simulink model "SymmetricInterpolationFIR"  (R2024a)
settings: Solver=VariableStepAuto  StartTime=0.0  StopTime=300E-9  RelTol=1e-3
InitFcn:
  | coef=[-58,15,80,95,52,-27,-89,-96,-43,38,97,95,32,-53,-104,-90,-18,67,109,83,1,-80,-111,-69,16,94,109,54,-38,-106,-104,-32,62,117,95,7,-89,-127,-80,23,117,134,60,-60,-148,-139,-35,102,179,140,1,-150,-213,-137,38,205,249,130,-89,-269,-286,-117,146,337,323,97,-216,-415,-362,-69,295,501,402,34,-390,-598,-440,13,497,704,479,-71,-621,-824,-517,143,766,955,554,-232,-935,-1106,-589,341,1132,1275,623,-477,-1369,-1472,-655,646,1652,1703,683,-859,-2000,-1983,-710,1134,2441,2334,734,-1501,-3026,-2794,-756,2016,3845,3445,771,-2793,-5097,-4460,-785,4114,7301,6322,795,-6901,-12353,-11074,-800,17016,37340,53412,59511,53412,37340,17016,-800,-11074,-12353,-6901,795,6322,7301,4114,-785,-4460,-5097,-2793,771,3445,3845,2016,-756,-2794,-3026,-1501,734,2334,2441,1134,-710,-1983,-2000,-859,683,1703,1652,646,-655,-1472,-1369,-477,623,1275,1132,341,-589,-1106,-935,-232,554,955,766,143,-517,-824,-621,-71,479,704,497,13,-440,-598,-390,34,402,501,295,-69,-362,-415,-216,97,323,337,146,-117,-286,-269,-89,130,249,205,38,-137,-213,-150,1,140,179,102,-35,-139,-148,-60,60,134,117,23,-80,-127,-89,7,95,117,62,-32,-104,-106,-38,54,109,94,16,-69,-111,-80,1,83,109,67,-18,-90,-104,-53,32,95,97,38,-43,-96,-89,-27,52,95,80,15,-58;
  |        10,35,36,11,-23,-40,-29,4,35,41,18,-20,-45,-39,-4,36,52,31,-13,-51,-54,-20,31,63,52,5,-48,-69,-43,14,63,69,28,-33,-73,-62,-7,52,76,46,-17,-69,-72,-23,45,81,59,-8,-73,-87,-36,45,98,83,4,-85,-119,-69,35,123,131,45,-80,-158,-131,-10,126,183,117,-34,-168,-193,-86,85,202,183,36,-140,-220,-145,34,193,214,76,-124,-239,-176,30,233,272,97,-181,-359,-280,35,382,498,254,-232,-638,-648,-181,507,958,803,46,-881,-1353,-958,175,1383,1842,1107,-514,-2062,-2461,-1246,1032,3006,3282,1368,-1842,-4413,-4475,-1468,3226,6794,6517,1542,-6108,-12043,-11443,-1589,16342,37236,53942,60315,53942,37236,16342,-1589,-11443,-12043,-6108,1542,6517,6794,3226,-1468,-4475,-4413,-1842,1368,3282,3006,1032,-1246,-2461,-2062,-514,1107,1842,1383,175,-958,-1353,-881,46,803,958,507,-181,-648,-638,-232,254,498,382,35,-280,-359,-181,97,272,233,30,-176,-239,-124,76,214,193,34,-145,-220,-140,36,183,202,85,-86,-193,-168,-34,117,183,126,-10,-131,-158,-80,45,131,123,35,-69,-119,-85,4,83,98,45,-36,-87,-73,-8,59,81,45,-23,-72,-69,-17,46,76,52,-7,-62,-73,-33,28,69,63,14,-43,-69,-48,5,52,63,31,-20,-54,-51,-13,31,52,36,-4,-39,-45,-20,18,41,35,4,-29,-40,-23,11,36,35,10;
  |        25,21,1,-21,-29,-13,13,31,25,1,-25,-33,-16,13,33,28,2,-26,-35,-16,15,35,28,-2,-31,-36,-13,21,42,30,-7,-40,-45,-15,28,52,37,-6,-47,-53,-21,29,57,42,-5,-49,-55,-19,35,62,40,-15,-61,-61,-11,51,78,46,-26,-84,-81,-16,66,103,64,-24,-99,-101,-28,68,115,73,-26,-106,-104,-18,88,128,63,-60,-147,-122,7,149,188,83,-103,-231,-197,-7,205,284,155,-98,-293,-278,-53,220,332,186,-115,-335,-284,22,350,410,104,-376,-641,-403,264,904,972,253,-885,-1644,-1322,120,1866,2662,1662,-852,-3402,-4110,-1964,2238,6000,6443,2202,-5207,-11536,-11669,-2354,15609,37069,54456,61128,54456,37069,15609,-2354,-11669,-11536,-5207,2202,6443,6000,2238,-1964,-4110,-3402,-852,1662,2662,1866,120,-1322,-1644,-885,253,972,904,264,-403,-641,-376,104,410,350,22,-284,-335,-115,186,332,220,-53,-278,-293,-98,155,284,205,-7,-197,-231,-103,83,188,149,7,-122,-147,-60,63,128,88,-18,-104,-106,-26,73,115,68,-28,-101,-99,-24,64,103,66,-16,-81,-84,-26,46,78,51,-11,-61,-61,-15,40,62,35,-19,-55,-49,-5,42,57,29,-21,-53,-47,-6,37,52,28,-15,-45,-40,-7,30,42,21,-13,-36,-31,-2,28,35,15,-16,-35,-26,2,28,33,13,-16,-33,-25,1,25,31,13,-13,-29,-21,1,21,25;
  |        17,0,-17,-21,-8,12,22,14,-7,-21,-19,0,19,23,7,-16,-26,-15,9,27,24,0,-24,-29,-10,17,31,20,-9,-29,-26,0,27,32,9,-23,-38,-22,14,40,34,0,-36,-43,-16,26,46,29,-12,-44,-40,0,42,49,14,-36,-59,-33,23,64,55,0,-59,-72,-27,41,77,50,-20,-74,-66,0,70,83,23,-64,-105,-59,43,120,104,0,-112,-140,-56,77,151,102,-34,-146,-133,0,146,172,43,-149,-237,-129,114,301,262,0,-296,-385,-171,197,427,316,-69,-411,-400,0,466,552,76,-654,-997,-482,716,1743,1607,0,-2228,-3420,-2217,1249,4986,6105,2736,-4234,-10850,-11747,-3086,14817,36834,54947,61945,54947,36834,14817,-3086,-11747,-10850,-4234,2736,6105,4986,1249,-2217,-3420,-2228,0,1607,1743,716,-482,-997,-654,76,552,466,0,-400,-411,-69,316,427,197,-171,-385,-296,0,262,301,114,-129,-237,-149,43,172,146,0,-133,-146,-34,102,151,77,-56,-140,-112,0,104,120,43,-59,-105,-64,23,83,70,0,-66,-74,-20,50,77,41,-27,-72,-59,0,55,64,23,-33,-59,-36,14,49,42,0,-40,-44,-12,29,46,26,-16,-43,-36,0,34,40,14,-22,-38,-23,9,32,27,0,-26,-29,-9,20,31,17,-10,-29,-24,0,24,27,9,-15,-26,-16,7,23,19,0,-19,-21,-7,14,22,12,-8,-21,-17,0,17];
  | coef=coef';
  | H0=coef(1:4:273,:);H0=H0(:);
  | H1=coef(2:4:273,:);H1=H1(:);
  | H2=coef(3:4:273,:);H2=H2(:);
  | H3=coef(4:4:273,:);H3=H3(:);
  | H1PH3=H1+H3;
  | H1MH3=H1-H3;
undefined symbols (not defined in the file): S, vsva2197, xcvc1902
libraries: hdlBasic x29, hdlDSPIP x8, hdlUtilities x1, dspsrcs4 x1, dspsigops x1, vmcUtilities x1
settings Model: Creator=admin  LastModifiedBy=sdegala
settings SolverCC: AlgebraicLoopSolver=TrustRegion
settings DataIOCC: ReturnWorkspaceOutputs=off
settings DebuggingCC: UnconnectedInputMsg=warning  UnconnectedOutputMsg=warning  UnconnectedLineMsg=warning  ArithmeticOperatorsInVariantConditions=warning
settings ModelReferenceCC: EnableRefExpFcnMdlSchedulingChecks=on
settings SFSimCC: SimUseLocalCustomCode=off  CustomCodeUndefinedFunction=UseInterfaceOnly
settings RTWCC: RTWUseLocalCustomCode=off  GPUComputeCapability=3.5  DLArmComputeVersion=19.05
settings CodeAppCC: StateflowObjectComments=on

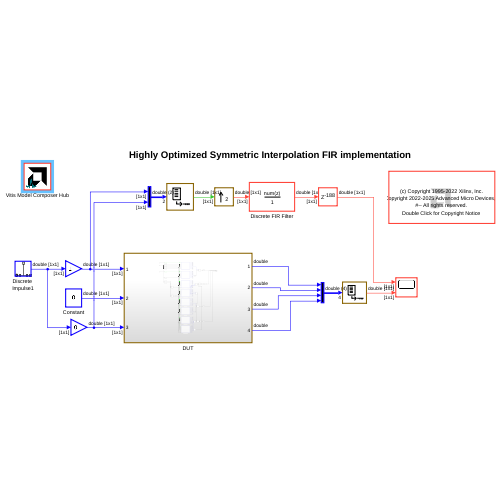
[thumbnail: Simulink's stored preview of the top-level diagram]
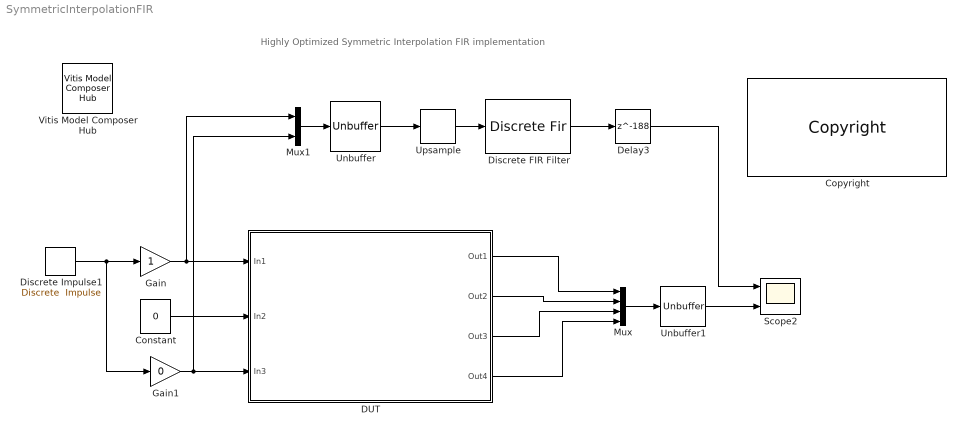
== system SymmetricInterpolationFIR ==
  note: Highly Optimized Symmetric Interpolation FIR implementation
  Constant : Constant  Value=0  VectorParams1D=off  SampleTime=-1
  Copyright : hdlUtilities/Copyright  copyrighttext="(c) Copyright 1995-2022 Xilinx, Inc. <br>(c) Copyright 2022-2025 Advanced Micro Devices, Inc. All rights reserved.<br><br>This document  contains proprietary, confidential information that may be used, copied and/or disclosed only as authorized by a valid licensing agreement with Advanced Micro Devices, Inc. This copyright notice must be retained on all authorized copies.<br><br> This code is provided \"as is\". Advanced Micro Devices, Inc. makes, and the end user receives, no warranties or conditions, express, implied, statutory or otherwise, and Advanced Micro Devices, Inc. specifically disclaims any implied warranties of merchantability, <br>non-infringement, or fitness for a particular purpose."  block_type=copyright
  DUT : Subsystem
  Delay3 : Delay  DelayLength=188
  Discrete Impulse1 : dspsrcs4/Discrete  Impulse  Delay=10  SampleTime=-1  FrameSample=1  OutputFrames=off  dataType=double  isSigned=on  wordLen=16  udDataType=sfix(16)  fracBitsMode=Best precision  numFracBits=15  OutDataTypeStr=double  LastOutDataTypeStr=double
  Discrete FIR Filter : DiscreteFir  Coefficients=coef(:,1)'  InputProcessing=Columns as channels (frame based)
  Gain : Gain
  Gain1 : Gain  Gain=0
  Mux : Mux
  Mux1 : Mux  Inputs=2
  Scope2 : Scope  NumInputPorts=2
  Unbuffer : Unbuffer
  Unbuffer1 : Unbuffer
  Upsample : dspsigops/Upsample  FactorSource=Dialog parameter  N=2  Nmax=16  phase=0  RateOptions=Allow multirate processing  ic=0  mode=Unused parameter value
  Vitis Model Composer Hub : vmcUtilities/Vitis Model Composer Hub  Tag=genX  CodeGeneration=off  SubsystemName=DUT  BlockHierPath=SymmetricInterpolationFIR/DUT  CompilationType=HDLCompilation  SubsystemType=HDLNode  ExportTypeV2=IP Catalog  StartColumn=1  NumberOfColumns=1  TargetDirectory=./netlist  exportDesign=on  analyzeDesign=off  validateDesignOnHw=off  ExportType=System Generator  IpVendor=xilinx.com  IpLibrary=hls  IpVersion=1.0  IpHWLanguage=Verilog  AieCompilerOptions={}  AieSimulatorOptions={}  CreateTestbench=off  TestbenchStackSize=10  RunRtlSim=off  RunCSim=off  RunAieSim=off  AieSimTimeout=50000  RunAieSimProfiling=off  LaunchVitisAnalyzer=off  PlotOutput=off  RunX86Sim=off  X86SimTimeout=10  GenHwImage=off  GenLibadfXo=off  GenHwValidationCode=off  PlatformType=Specify Platform  Platform=/proj/xbuilds/SWIP/9999.0_0905_1841/installs/lin64/2025.2/Vitis/base_platforms/xilinx_vck190_base_202520_1/xilinx_vck190_base_202520_1.xpfm  HwSystemType=Baremetal  HwValidationTarget=hw  ProjDevice=Versal VCK190 Evaluation Platform (xcvc1902-vsva2197-2MP-e-S)  ProjDevicePart=xcvc1902-vsva2197-2MP-e-S  AIEType=AIE  SamplePeriod=-1  ClockFrequency=200  DataPathParallelism=1  xilinxfamily=versalaicore  part=xcvc1902  speed=-2MP-e-S  package=vsva2197  directory=./netlist/ip/DUT/src  testbench=off  incr_netlist=off  synthesis_tool=Vivado  clock_wrapper=Clock Enables  dbl_ovrd=According to Block Masks  dcm_input_clock_period=10  sysclk_period=2  simulink_period=2E-9  eval_field=0  IPInfoJsonString="{\"DUTSubsystemName\":\"DUT\",\"HDLSubsystem\":{\"SubsystemName\":\"DUT\",\"IPName\":\"Subsystem\",\"IPLibrary\":\"VMC\",\"IPVendor\":\"User Company\",\"IPVersion\":\"1.0\",\"TargetDirectory\":\"./netlist\",\"SubsystemDir\":\"./netlist/ip/DUT\",\"FreqHz\":\"500000000\"},\"SubsystemTag\":\"HDLNode\"}"  LogFileName=/proj/xhdhdstaff5/sdegala/Head1/HEAD/ModelComposer_Sept16/Vitis_Model_Composer/Examples/HDL/RFSoC/Symmetric_Interpolation_FIR/netlist/model_composer.log  NThreads=4  IPConfigFile=/tmp/vmctmp-10925933730550270575/SymmetricInterpolationFIR_ipconfig.json
  wires:
  Discrete Impulse1/1 -> Gain1/1, Gain/1
  Mux/1 -> Unbuffer1/1
  Unbuffer1/1 -> Scope2/2
  Gain/1 -> Mux1/1, DUT/1(In1)
  Gain1/1 -> Mux1/2, DUT/3(In3)
  Upsample/1 -> Discrete FIR Filter/1
  Unbuffer/1 -> Upsample/1
  Mux1/1 -> Unbuffer/1
  Discrete FIR Filter/1 -> Delay3/1
  Delay3/1 -> Scope2/1
  Constant/1 -> DUT/2(In2)
  DUT/1(Out1) -> Mux/1
  DUT/2(Out2) -> Mux/2
  DUT/3(Out3) -> Mux/3
  DUT/4(Out4) -> Mux/4

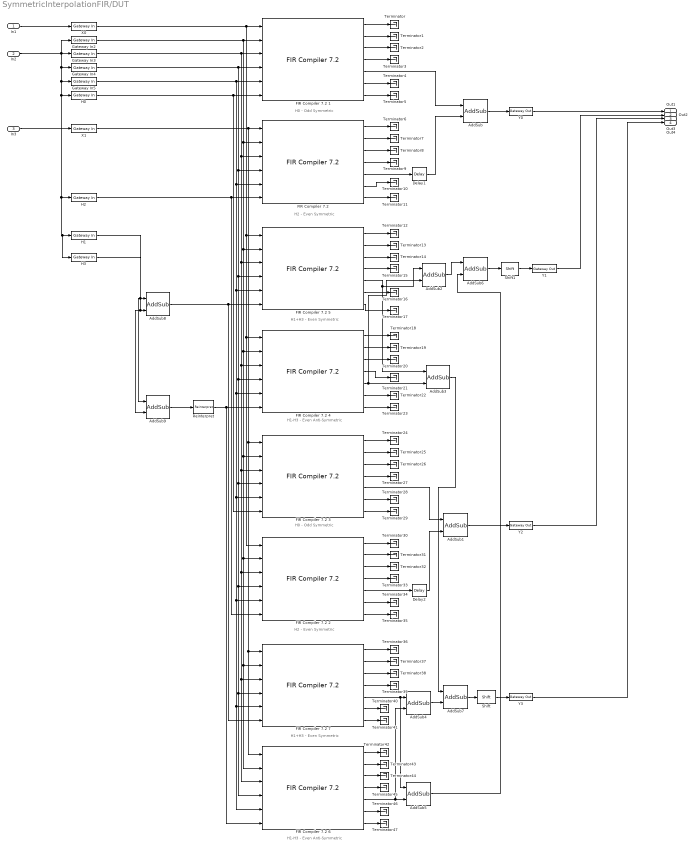
== system SymmetricInterpolationFIR/DUT ==
  note: H0 - Odd Symmetric
  note: H2 - Even Symmetric
  note: H2 - Even Symmetric
  note: H0 - Odd Symmetric
  note: H1-H3 - Even Anti-Symmetric
  note: H1+H3 - Even Symmetric
  note: H1-H3 - Even Anti-Symmetric
  note: H1+H3 - Even Symmetric
  In1 : Inport
  In2 : Inport  Port=2
  In3 : Inport  Port=3
  AddSub{,1..2,4,6..7} (6 alike) : hdlBasic/AddSub  mode=Addition  use_carryin=off  use_carryout=off  en=off  latency=1  precision=Full  arith_type=Unsigned  n_bits=16  bin_pt=14  quantization=Truncate  overflow=Wrap  use_behavioral_HDL=off  hw_selection=Fabric  pipelined=off  XmcBlockStatus=1  maskContainerNames=tabcontainer1  block_type=addsub  block_config=sysgen:Addsub_config
  AddSub3 : hdlBasic/AddSub  mode=Subtraction  use_carryin=off  use_carryout=off  en=off  latency=1  precision=Full  arith_type=Unsigned  n_bits=16  bin_pt=14  quantization=Truncate  overflow=Wrap  use_behavioral_HDL=off  hw_selection=Fabric  pipelined=off  XmcBlockStatus=1  maskContainerNames=tabcontainer1  block_type=addsub  block_config=sysgen:Addsub_config
  AddSub5 : hdlBasic/AddSub  mode=Subtraction  use_carryin=off  use_carryout=off  en=off  latency=2  precision=Full  arith_type=Unsigned  n_bits=16  bin_pt=14  quantization=Truncate  overflow=Wrap  use_behavioral_HDL=off  hw_selection=Fabric  pipelined=off  XmcBlockStatus=1  maskContainerNames=tabcontainer1  block_type=addsub  block_config=sysgen:Addsub_config
  AddSub8 : hdlBasic/AddSub  mode=Addition  use_carryin=off  use_carryout=off  en=off  latency=0  precision=Full  arith_type=Unsigned  n_bits=18  bin_pt=0  quantization=Truncate  overflow=Wrap  use_behavioral_HDL=off  hw_selection=Fabric  pipelined=off  XmcBlockStatus=1  maskContainerNames=tabcontainer1  block_type=addsub  block_config=sysgen:Addsub_config
  AddSub9 : hdlBasic/AddSub  mode=Subtraction  use_carryin=off  use_carryout=off  en=off  latency=0  precision=Full  arith_type=Unsigned  n_bits=18  bin_pt=0  quantization=Truncate  overflow=Wrap  use_behavioral_HDL=off  hw_selection=Fabric  pipelined=off  XmcBlockStatus=1  maskContainerNames=tabcontainer1  block_type=addsub  block_config=sysgen:Addsub_config
  Delay1 : hdlBasic/Delay  rst=off  en=off  latency=2  reg_retiming=off  XmcBlockStatus=1  maskContainerNames=group1  block_type=delay  block_config=sysgen:Delay_config
  Delay2 : hdlBasic/Delay  rst=off  en=off  latency=1  reg_retiming=off  XmcBlockStatus=1  maskContainerNames=group1  block_type=delay  block_config=sysgen:Delay_config
  "FIR Compiler 7.2 " : hdlDSPIP/FIR Compiler 7.2   coefficientvector=H2  coefficient_sets=4  coefficient_reload=on  filter_type=Single_Rate  rate_change_type=Integer  interpolation_rate=1  decimation_rate=1  zero_pack_factor=1  channel_sequence=Basic  number_channels=1  pattern_list='P4-0,P4-1,P4-2,P4-3,P4-4'  number_paths=1  ratespecification=Maximum_Possible  sampleperiod=0.33333333  hardwareoversamplingrate=1  coefficient_sign=Signed  quantization=Integer_Coefficients  coefficient_width=17  bestprecision=off  coefficient_fractional_bits=0  coefficient_structure=Symmetric  output_rounding_mode=Full_Precision  output_width=40  filter_architecture=Systolic_Multiply_Accumulate  optimization_goal=Area  optimization_list='None'  data_buffer_type=Automatic  coefficient_buffer_type=Automatic  input_buffer_type=Automatic  output_buffer_type=Automatic  preference_for_other_storage=Automatic  multi_column_support=Automatic  columnconfig='34'  inter_column_pipe_length=4  data_has_tlast=Not_Required  m_data_has_tready=off  s_data_has_fifo=off  s_data_has_tuser=Not_Required  m_data_has_tuser=Not_Required  s_config_sync_mode=On_Vector  s_config_method=Single  num_reload_slots=1  has_aclken=off  has_aresetn=off  reset_data_vector=on  trim_axipin_name=on  simulation_type=hybrid_sim  simulation_model=sysgen:xfirv7_2_cmodel  data_path_portlist={ 's_axis_data_tdata', 'm_axis_data_tdata' }  passband_min=0.0  passband_max=0.5  stopband_min=0.5  stopband_max=1.0  filter_selection=1  gui_behaviour='Sysgen_GUI'  data_sign=Signed  data_width=16  data_fractional_bits=0  data_tuser_width=1  wrapper_available=true  ip_wrap_arbitrary_binary_point=true  ip_name=FIR Compiler  ip_version=7.2  dsptool_ready=true  ipcore_usecache=true  ipcore_useipmodelcache=true  port_translation_map={ 'aclken' => 'en', 'aresetn' => 'rst' }  run_core_at_system_period=true  ipcore_xco_need_fpga_part=true  ipcore_fpga_part=[]  XmcBlockStatus=1  maskContainerNames=tabcontainer1  block_type=fir_compiler_v7_2  block_config=sysgen:rodinimport_config  block_width=820  block_height=600
  FIR Compiler 7.2 1 : hdlDSPIP/FIR Compiler 7.2   coefficientvector=H0  coefficient_sets=4  coefficient_reload=on  filter_type=Single_Rate  rate_change_type=Integer  interpolation_rate=1  decimation_rate=1  zero_pack_factor=1  channel_sequence=Basic  number_channels=1  pattern_list='P4-0,P4-1,P4-2,P4-3,P4-4'  number_paths=1  ratespecification=Maximum_Possible  sampleperiod=0.33333333  hardwareoversamplingrate=1  coefficient_sign=Signed  quantization=Integer_Coefficients  coefficient_width=17  bestprecision=off  coefficient_fractional_bits=0  coefficient_structure=Symmetric  output_rounding_mode=Full_Precision  output_width=40  filter_architecture=Systolic_Multiply_Accumulate  optimization_goal=Area  optimization_list='None'  data_buffer_type=Automatic  coefficient_buffer_type=Automatic  input_buffer_type=Automatic  output_buffer_type=Automatic  preference_for_other_storage=Automatic  multi_column_support=Automatic  columnconfig='35'  inter_column_pipe_length=4  data_has_tlast=Not_Required  m_data_has_tready=off  s_data_has_fifo=off  s_data_has_tuser=Not_Required  m_data_has_tuser=Not_Required  s_config_sync_mode=On_Vector  s_config_method=Single  num_reload_slots=1  has_aclken=off  has_aresetn=off  reset_data_vector=on  trim_axipin_name=on  simulation_type=hybrid_sim  simulation_model=sysgen:xfirv7_2_cmodel  data_path_portlist={ 's_axis_data_tdata', 'm_axis_data_tdata' }  passband_min=0.0  passband_max=0.5  stopband_min=0.5  stopband_max=1.0  filter_selection=1  gui_behaviour='Sysgen_GUI'  data_sign=Signed  data_width=16  data_fractional_bits=0  data_tuser_width=1  wrapper_available=true  ip_wrap_arbitrary_binary_point=true  ip_name=FIR Compiler  ip_version=7.2  dsptool_ready=true  ipcore_usecache=true  ipcore_useipmodelcache=true  port_translation_map={ 'aclken' => 'en', 'aresetn' => 'rst' }  run_core_at_system_period=true  ipcore_xco_need_fpga_part=true  ipcore_fpga_part=[]  XmcBlockStatus=1  maskContainerNames=tabcontainer1  block_type=fir_compiler_v7_2  block_config=sysgen:rodinimport_config  block_width=820  block_height=600
  FIR Compiler 7.2 2 : hdlDSPIP/FIR Compiler 7.2   coefficientvector=H2  coefficient_sets=4  coefficient_reload=on  filter_type=Single_Rate  rate_change_type=Integer  interpolation_rate=1  decimation_rate=1  zero_pack_factor=1  channel_sequence=Basic  number_channels=1  pattern_list='P4-0,P4-1,P4-2,P4-3,P4-4'  number_paths=1  ratespecification=Maximum_Possible  sampleperiod=0.33333333  hardwareoversamplingrate=1  coefficient_sign=Signed  quantization=Integer_Coefficients  coefficient_width=17  bestprecision=off  coefficient_fractional_bits=0  coefficient_structure=Symmetric  output_rounding_mode=Full_Precision  output_width=40  filter_architecture=Systolic_Multiply_Accumulate  optimization_goal=Area  optimization_list='None'  data_buffer_type=Automatic  coefficient_buffer_type=Automatic  input_buffer_type=Automatic  output_buffer_type=Automatic  preference_for_other_storage=Automatic  multi_column_support=Automatic  columnconfig='34'  inter_column_pipe_length=4  data_has_tlast=Not_Required  m_data_has_tready=off  s_data_has_fifo=off  s_data_has_tuser=Not_Required  m_data_has_tuser=Not_Required  s_config_sync_mode=On_Vector  s_config_method=Single  num_reload_slots=1  has_aclken=off  has_aresetn=off  reset_data_vector=on  trim_axipin_name=on  simulation_type=hybrid_sim  simulation_model=sysgen:xfirv7_2_cmodel  data_path_portlist={ 's_axis_data_tdata', 'm_axis_data_tdata' }  passband_min=0.0  passband_max=0.5  stopband_min=0.5  stopband_max=1.0  filter_selection=1  gui_behaviour='Sysgen_GUI'  data_sign=Signed  data_width=16  data_fractional_bits=0  data_tuser_width=1  wrapper_available=true  ip_wrap_arbitrary_binary_point=true  ip_name=FIR Compiler  ip_version=7.2  dsptool_ready=true  ipcore_usecache=true  ipcore_useipmodelcache=true  port_translation_map={ 'aclken' => 'en', 'aresetn' => 'rst' }  run_core_at_system_period=true  ipcore_xco_need_fpga_part=true  ipcore_fpga_part=[]  XmcBlockStatus=1  maskContainerNames=tabcontainer1  block_type=fir_compiler_v7_2  block_config=sysgen:rodinimport_config  block_width=820  block_height=600
  FIR Compiler 7.2 3 : hdlDSPIP/FIR Compiler 7.2   coefficientvector=H0  coefficient_sets=4  coefficient_reload=on  filter_type=Single_Rate  rate_change_type=Integer  interpolation_rate=1  decimation_rate=1  zero_pack_factor=1  channel_sequence=Basic  number_channels=1  pattern_list='P4-0,P4-1,P4-2,P4-3,P4-4'  number_paths=1  ratespecification=Maximum_Possible  sampleperiod=0.33333333  hardwareoversamplingrate=1  coefficient_sign=Signed  quantization=Integer_Coefficients  coefficient_width=17  bestprecision=off  coefficient_fractional_bits=0  coefficient_structure=Symmetric  output_rounding_mode=Full_Precision  output_width=40  filter_architecture=Systolic_Multiply_Accumulate  optimization_goal=Area  optimization_list='None'  data_buffer_type=Automatic  coefficient_buffer_type=Automatic  input_buffer_type=Automatic  output_buffer_type=Automatic  preference_for_other_storage=Automatic  multi_column_support=Automatic  columnconfig='35'  inter_column_pipe_length=4  data_has_tlast=Not_Required  m_data_has_tready=off  s_data_has_fifo=off  s_data_has_tuser=Not_Required  m_data_has_tuser=Not_Required  s_config_sync_mode=On_Vector  s_config_method=Single  num_reload_slots=1  has_aclken=off  has_aresetn=off  reset_data_vector=on  trim_axipin_name=on  simulation_type=hybrid_sim  simulation_model=sysgen:xfirv7_2_cmodel  data_path_portlist={ 's_axis_data_tdata', 'm_axis_data_tdata' }  passband_min=0.0  passband_max=0.5  stopband_min=0.5  stopband_max=1.0  filter_selection=1  gui_behaviour='Sysgen_GUI'  data_sign=Signed  data_width=16  data_fractional_bits=0  data_tuser_width=1  wrapper_available=true  ip_wrap_arbitrary_binary_point=true  ip_name=FIR Compiler  ip_version=7.2  dsptool_ready=true  ipcore_usecache=true  ipcore_useipmodelcache=true  port_translation_map={ 'aclken' => 'en', 'aresetn' => 'rst' }  run_core_at_system_period=true  ipcore_xco_need_fpga_part=true  ipcore_fpga_part=[]  XmcBlockStatus=1  maskContainerNames=tabcontainer1  block_type=fir_compiler_v7_2  block_config=sysgen:rodinimport_config  block_width=820  block_height=600
  FIR Compiler 7.2 4 : hdlDSPIP/FIR Compiler 7.2   coefficientvector=H1MH3  coefficient_sets=4  coefficient_reload=on  filter_type=Single_Rate  rate_change_type=Integer  interpolation_rate=1  decimation_rate=1  zero_pack_factor=1  channel_sequence=Basic  number_channels=1  pattern_list='P4-0,P4-1,P4-2,P4-3,P4-4'  number_paths=1  ratespecification=Maximum_Possible  sampleperiod=0.33333333  hardwareoversamplingrate=1  coefficient_sign=Signed  quantization=Integer_Coefficients  coefficient_width=18  bestprecision=off  coefficient_fractional_bits=0  coefficient_structure=Negative_Symmetric  output_rounding_mode=Full_Precision  output_width=41  filter_architecture=Systolic_Multiply_Accumulate  optimization_goal=Area  optimization_list='None'  data_buffer_type=Automatic  coefficient_buffer_type=Automatic  input_buffer_type=Automatic  output_buffer_type=Automatic  preference_for_other_storage=Automatic  multi_column_support=Automatic  columnconfig='34'  inter_column_pipe_length=4  data_has_tlast=Not_Required  m_data_has_tready=off  s_data_has_fifo=off  s_data_has_tuser=Not_Required  m_data_has_tuser=Not_Required  s_config_sync_mode=On_Vector  s_config_method=Single  num_reload_slots=1  has_aclken=off  has_aresetn=off  reset_data_vector=on  trim_axipin_name=on  simulation_type=hybrid_sim  simulation_model=sysgen:xfirv7_2_cmodel  data_path_portlist={ 's_axis_data_tdata', 'm_axis_data_tdata' }  passband_min=0.0  passband_max=0.5  stopband_min=0.5  stopband_max=1.0  filter_selection=1  gui_behaviour='Sysgen_GUI'  data_sign=Signed  data_width=16  data_fractional_bits=0  data_tuser_width=1  wrapper_available=true  ip_wrap_arbitrary_binary_point=true  ip_name=FIR Compiler  ip_version=7.2  dsptool_ready=true  ipcore_usecache=true  ipcore_useipmodelcache=true  port_translation_map={ 'aclken' => 'en', 'aresetn' => 'rst' }  run_core_at_system_period=true  ipcore_xco_need_fpga_part=true  ipcore_fpga_part=[]  XmcBlockStatus=1  maskContainerNames=tabcontainer1  block_type=fir_compiler_v7_2  block_config=sysgen:rodinimport_config  block_width=820  block_height=600
  FIR Compiler 7.2 5 : hdlDSPIP/FIR Compiler 7.2   coefficientvector=H1PH3  coefficient_sets=4  coefficient_reload=on  filter_type=Single_Rate  rate_change_type=Integer  interpolation_rate=1  decimation_rate=1  zero_pack_factor=1  channel_sequence=Basic  number_channels=1  pattern_list='P4-0,P4-1,P4-2,P4-3,P4-4'  number_paths=1  ratespecification=Maximum_Possible  sampleperiod=0.33333333  hardwareoversamplingrate=1  coefficient_sign=Signed  quantization=Integer_Coefficients  coefficient_width=18  bestprecision=off  coefficient_fractional_bits=0  coefficient_structure=Symmetric  output_rounding_mode=Full_Precision  output_width=41  filter_architecture=Systolic_Multiply_Accumulate  optimization_goal=Area  optimization_list='None'  data_buffer_type=Automatic  coefficient_buffer_type=Automatic  input_buffer_type=Automatic  output_buffer_type=Automatic  preference_for_other_storage=Automatic  multi_column_support=Automatic  columnconfig='34'  inter_column_pipe_length=4  data_has_tlast=Not_Required  m_data_has_tready=off  s_data_has_fifo=off  s_data_has_tuser=Not_Required  m_data_has_tuser=Not_Required  s_config_sync_mode=On_Vector  s_config_method=Single  num_reload_slots=1  has_aclken=off  has_aresetn=off  reset_data_vector=on  trim_axipin_name=on  simulation_type=hybrid_sim  simulation_model=sysgen:xfirv7_2_cmodel  data_path_portlist={ 's_axis_data_tdata', 'm_axis_data_tdata' }  passband_min=0.0  passband_max=0.5  stopband_min=0.5  stopband_max=1.0  filter_selection=1  gui_behaviour='Sysgen_GUI'  data_sign=Signed  data_width=16  data_fractional_bits=0  data_tuser_width=1  wrapper_available=true  ip_wrap_arbitrary_binary_point=true  ip_name=FIR Compiler  ip_version=7.2  dsptool_ready=true  ipcore_usecache=true  ipcore_useipmodelcache=true  port_translation_map={ 'aclken' => 'en', 'aresetn' => 'rst' }  run_core_at_system_period=true  ipcore_xco_need_fpga_part=true  ipcore_fpga_part=[]  XmcBlockStatus=1  maskContainerNames=tabcontainer1  block_type=fir_compiler_v7_2  block_config=sysgen:rodinimport_config  block_width=820  block_height=600
  FIR Compiler 7.2 6 : hdlDSPIP/FIR Compiler 7.2   coefficientvector=H1MH3  coefficient_sets=4  coefficient_reload=on  filter_type=Single_Rate  rate_change_type=Integer  interpolation_rate=1  decimation_rate=1  zero_pack_factor=1  channel_sequence=Basic  number_channels=1  pattern_list='P4-0,P4-1,P4-2,P4-3,P4-4'  number_paths=1  ratespecification=Maximum_Possible  sampleperiod=0.33333333  hardwareoversamplingrate=1  coefficient_sign=Signed  quantization=Integer_Coefficients  coefficient_width=18  bestprecision=off  coefficient_fractional_bits=0  coefficient_structure=Negative_Symmetric  output_rounding_mode=Full_Precision  output_width=41  filter_architecture=Systolic_Multiply_Accumulate  optimization_goal=Area  optimization_list='None'  data_buffer_type=Automatic  coefficient_buffer_type=Automatic  input_buffer_type=Automatic  output_buffer_type=Automatic  preference_for_other_storage=Automatic  multi_column_support=Automatic  columnconfig='34'  inter_column_pipe_length=4  data_has_tlast=Not_Required  m_data_has_tready=off  s_data_has_fifo=off  s_data_has_tuser=Not_Required  m_data_has_tuser=Not_Required  s_config_sync_mode=On_Vector  s_config_method=Single  num_reload_slots=1  has_aclken=off  has_aresetn=off  reset_data_vector=on  trim_axipin_name=on  simulation_type=hybrid_sim  simulation_model=sysgen:xfirv7_2_cmodel  data_path_portlist={ 's_axis_data_tdata', 'm_axis_data_tdata' }  passband_min=0.0  passband_max=0.5  stopband_min=0.5  stopband_max=1.0  filter_selection=1  gui_behaviour='Sysgen_GUI'  data_sign=Signed  data_width=16  data_fractional_bits=0  data_tuser_width=1  wrapper_available=true  ip_wrap_arbitrary_binary_point=true  ip_name=FIR Compiler  ip_version=7.2  dsptool_ready=true  ipcore_usecache=true  ipcore_useipmodelcache=true  port_translation_map={ 'aclken' => 'en', 'aresetn' => 'rst' }  run_core_at_system_period=true  ipcore_xco_need_fpga_part=true  ipcore_fpga_part=[]  XmcBlockStatus=1  maskContainerNames=tabcontainer1  block_type=fir_compiler_v7_2  block_config=sysgen:rodinimport_config  block_width=820  block_height=600
  FIR Compiler 7.2 7 : hdlDSPIP/FIR Compiler 7.2   coefficientvector=H1PH3  coefficient_sets=4  coefficient_reload=on  filter_type=Single_Rate  rate_change_type=Integer  interpolation_rate=1  decimation_rate=1  zero_pack_factor=1  channel_sequence=Basic  number_channels=1  pattern_list='P4-0,P4-1,P4-2,P4-3,P4-4'  number_paths=1  ratespecification=Maximum_Possible  sampleperiod=0.33333333  hardwareoversamplingrate=1  coefficient_sign=Signed  quantization=Integer_Coefficients  coefficient_width=18  bestprecision=off  coefficient_fractional_bits=0  coefficient_structure=Symmetric  output_rounding_mode=Full_Precision  output_width=41  filter_architecture=Systolic_Multiply_Accumulate  optimization_goal=Area  optimization_list='None'  data_buffer_type=Automatic  coefficient_buffer_type=Automatic  input_buffer_type=Automatic  output_buffer_type=Automatic  preference_for_other_storage=Automatic  multi_column_support=Automatic  columnconfig='34'  inter_column_pipe_length=4  data_has_tlast=Not_Required  m_data_has_tready=off  s_data_has_fifo=off  s_data_has_tuser=Not_Required  m_data_has_tuser=Not_Required  s_config_sync_mode=On_Vector  s_config_method=Single  num_reload_slots=1  has_aclken=off  has_aresetn=off  reset_data_vector=on  trim_axipin_name=on  simulation_type=hybrid_sim  simulation_model=sysgen:xfirv7_2_cmodel  data_path_portlist={ 's_axis_data_tdata', 'm_axis_data_tdata' }  passband_min=0.0  passband_max=0.5  stopband_min=0.5  stopband_max=1.0  filter_selection=1  gui_behaviour='Sysgen_GUI'  data_sign=Signed  data_width=16  data_fractional_bits=0  data_tuser_width=1  wrapper_available=true  ip_wrap_arbitrary_binary_point=true  ip_name=FIR Compiler  ip_version=7.2  dsptool_ready=true  ipcore_usecache=true  ipcore_useipmodelcache=true  port_translation_map={ 'aclken' => 'en', 'aresetn' => 'rst' }  run_core_at_system_period=true  ipcore_xco_need_fpga_part=true  ipcore_fpga_part=[]  XmcBlockStatus=1  maskContainerNames=tabcontainer1  block_type=fir_compiler_v7_2  block_config=sysgen:rodinimport_config  block_width=820  block_height=600
  Gateway In2 : hdlBasic/Gateway In  gui_display_data_type=Boolean  arith_type=Boolean  n_bits=16  bin_pt=14  preci_type=Single  exp_width=8  frac_width=24  rows=1  columns=1  quantization="Round  (unbiased: +/- Inf)"  overflow=Saturate  period=2E-9  UseAsADC=off  ADCChannel='1'  interface=None  automatic_assignment=on  address_offset=hex2dec('00')  intf_name=''  intf_description=''  default_value=0  timing_constraint=None  locs_specified=off  LOCs={}  io_standard={}  inherit_from_input=off  hdl_port=on  XmcBlockStatus=1  maskContainerNames=group4  block_type=gatewayin  block_config=sysgen:gateway_in_config  block_width_w=590  block_height_w=620  block_width=640  block_height=850
  Gateway In3 : hdlBasic/Gateway In  gui_display_data_type=Fixed-point  arith_type=Unsigned  n_bits=2  bin_pt=0  preci_type=Single  exp_width=8  frac_width=24  rows=1  columns=1  quantization="Round  (unbiased: +/- Inf)"  overflow=Saturate  period=2E-9  UseAsADC=off  ADCChannel='1'  interface=None  automatic_assignment=on  address_offset=hex2dec('00')  intf_name=''  intf_description=''  default_value=0  timing_constraint=None  locs_specified=off  LOCs={}  io_standard={}  inherit_from_input=off  hdl_port=on  XmcBlockStatus=1  maskContainerNames=group4  block_type=gatewayin  block_config=sysgen:gateway_in_config  block_width_w=590  block_height_w=620  block_width=640  block_height=850
  Gateway In4 : hdlBasic/Gateway In  gui_display_data_type=Boolean  arith_type=Boolean  n_bits=16  bin_pt=0  preci_type=Single  exp_width=8  frac_width=24  rows=1  columns=1  quantization="Round  (unbiased: +/- Inf)"  overflow=Saturate  period=2E-9  UseAsADC=off  ADCChannel='1'  interface=None  automatic_assignment=on  address_offset=hex2dec('00')  intf_name=''  intf_description=''  default_value=0  timing_constraint=None  locs_specified=off  LOCs={}  io_standard={}  inherit_from_input=off  hdl_port=on  XmcBlockStatus=1  maskContainerNames=group4  block_type=gatewayin  block_config=sysgen:gateway_in_config  block_width_w=590  block_height_w=620  block_width=640  block_height=850
  Gateway In5 : hdlBasic/Gateway In  gui_display_data_type=Boolean  arith_type=Boolean  n_bits=16  bin_pt=0  preci_type=Single  exp_width=8  frac_width=24  rows=1  columns=1  quantization="Round  (unbiased: +/- Inf)"  overflow=Saturate  period=2E-9  UseAsADC=off  ADCChannel='1'  interface=None  automatic_assignment=on  address_offset=hex2dec('00')  intf_name=''  intf_description=''  default_value=0  timing_constraint=None  locs_specified=off  LOCs={}  io_standard={}  inherit_from_input=off  hdl_port=on  XmcBlockStatus=1  maskContainerNames=group4  block_type=gatewayin  block_config=sysgen:gateway_in_config  block_width_w=590  block_height_w=620  block_width=640  block_height=850
  H{0..3} (4 alike) : hdlBasic/Gateway In  gui_display_data_type=Fixed-point  arith_type=Unsigned  n_bits=17  bin_pt=0  preci_type=Single  exp_width=8  frac_width=24  rows=1  columns=1  quantization="Round  (unbiased: +/- Inf)"  overflow=Saturate  period=2E-9  UseAsADC=off  ADCChannel='1'  interface=None  automatic_assignment=on  address_offset=hex2dec('00')  intf_name=''  intf_description=''  default_value=0  timing_constraint=None  locs_specified=off  LOCs={}  io_standard={}  inherit_from_input=off  hdl_port=on  XmcBlockStatus=1  maskContainerNames=group4  block_type=gatewayin  block_config=sysgen:gateway_in_config  block_width_w=590  block_height_w=620  block_width=640  block_height=850
  Reinterpret : hdlBasic/Reinterpret  force_arith_type=on  arith_type=Unsigned  force_bin_pt=off  bin_pt=0  XmcBlockStatus=1  maskContainerNames=group1  block_type=reinterpret  block_config=sysgen:Reinterpret_config
  Shift : hdlBasic/Shift  shift_dir=Right  shift_bits=1  en=off  latency=0  precision=User Defined  arith_type="Signed  (2's comp)"  n_bits=41  bin_pt=0  quantization=Truncate  overflow=Wrap  XmcBlockStatus=1  maskContainerNames=group2  block_type=shift  block_config=sysgen:Shift_config
  Shift1 : hdlBasic/Shift  shift_dir=Right  shift_bits=1  en=off  latency=0  precision=User Defined  arith_type="Signed  (2's comp)"  n_bits=41  bin_pt=0  quantization=Truncate  overflow=Wrap  XmcBlockStatus=1  maskContainerNames=group2  block_type=shift  block_config=sysgen:Shift_config
  Terminator{,1..47} (48 alike) : Terminator
  X0 : hdlBasic/Gateway In  gui_display_data_type=Fixed-point  arith_type=Signed (2's comp)  n_bits=16  bin_pt=0  preci_type=Single  exp_width=8  frac_width=24  rows=1  columns=1  quantization="Round  (unbiased: +/- Inf)"  overflow=Saturate  period=2E-9  UseAsADC=off  ADCChannel='1'  interface=None  automatic_assignment=on  address_offset=hex2dec('00')  intf_name=''  intf_description=''  default_value=0  timing_constraint=None  locs_specified=off  LOCs={}  io_standard={}  inherit_from_input=off  hdl_port=on  XmcBlockStatus=1  maskContainerNames=group4  block_type=gatewayin  block_config=sysgen:gateway_in_config  block_width_w=590  block_height_w=620  block_width=640  block_height=850
  X1 : hdlBasic/Gateway In  gui_display_data_type=Fixed-point  arith_type=Signed (2's comp)  n_bits=16  bin_pt=0  preci_type=Single  exp_width=8  frac_width=24  rows=1  columns=1  quantization="Round  (unbiased: +/- Inf)"  overflow=Saturate  period=2E-9  UseAsADC=off  ADCChannel='1'  interface=None  automatic_assignment=on  address_offset=hex2dec('00')  intf_name=''  intf_description=''  default_value=0  timing_constraint=None  locs_specified=off  LOCs={}  io_standard={}  inherit_from_input=off  hdl_port=on  XmcBlockStatus=1  maskContainerNames=group4  block_type=gatewayin  block_config=sysgen:gateway_in_config  block_width_w=590  block_height_w=620  block_width=640  block_height=850
  Y{0..3} (4 alike) : hdlBasic/Gateway Out  inherit_from_input=off  bool_to_boolean=off  hdl_port=on  rows=1  columns=1  UseAsDAC=off  DACChannel='1'  interface=None  automatic_assignment=on  address_offset=hex2dec('00')  intf_name=''  intf_description=''  timing_constraint=None  locs_specified=off  LOCs={}  io_standard={}  XmcBlockStatus=1  maskContainerNames=group4  block_type=gatewayout  block_config=sysgen:gateway_out_config  block_width_w=590  block_height_w=620  block_width=620  block_height=750
  Out1 : Outport
  Out2 : Outport  Port=2
  Out3 : Outport  Port=3
  Out4 : Outport  Port=4
  wires:
  FIR Compiler 7.2 4/1 -> Terminator18/1
  FIR Compiler 7.2 7/1 -> Terminator36/1
  FIR Compiler 7.2 6/3 -> Terminator44/1
  AddSub3/1 -> AddSub7/1
  FIR Compiler 7.2 1/3 -> Terminator2/1
  Y1/1 -> Out2/1
  AddSub5/1 -> AddSub6/2
  FIR Compiler 7.2 1/2 -> Terminator1/1
  Gateway In2/1 -> FIR Compiler 7.2 1/2, FIR Compiler 7.2 5/2, FIR Compiler 7.2 4/2, FIR Compiler 7.2 3/2, FIR Compiler 7.2 7/2, FIR Compiler 7.2 6/2, FIR Compiler 7.2 2/2, "FIR Compiler 7.2 "/2
  Shift1/1 -> Y1/1
  In1/1 -> X0/1
  FIR Compiler 7.2 1/6 -> Terminator4/1
  FIR Compiler 7.2 5/2 -> Terminator13/1
  Gateway In4/1 -> FIR Compiler 7.2 1/4, "FIR Compiler 7.2 "/4, FIR Compiler 7.2 5/4, FIR Compiler 7.2 4/4, FIR Compiler 7.2 3/4, FIR Compiler 7.2 7/4, FIR Compiler 7.2 6/4, FIR Compiler 7.2 2/4
  FIR Compiler 7.2 5/5 -> AddSub3/1, AddSub2/1
  FIR Compiler 7.2 6/5 -> AddSub5/2, AddSub4/2
  FIR Compiler 7.2 6/6 -> Terminator46/1
  FIR Compiler 7.2 7/2 -> Terminator37/1
  AddSub7/1 -> Shift/1
  X1/1 -> FIR Compiler 7.2 6/1, FIR Compiler 7.2 7/1, FIR Compiler 7.2 3/1, "FIR Compiler 7.2 "/1
  FIR Compiler 7.2 7/7 -> Terminator41/1
  "FIR Compiler 7.2 "/1 -> Terminator6/1
  Gateway In3/1 -> FIR Compiler 7.2 1/3, FIR Compiler 7.2 5/3, FIR Compiler 7.2 4/3, FIR Compiler 7.2 3/3, FIR Compiler 7.2 7/3, FIR Compiler 7.2 6/3, FIR Compiler 7.2 2/3, "FIR Compiler 7.2 "/3
  FIR Compiler 7.2 7/5 -> AddSub5/1, AddSub4/1
  "FIR Compiler 7.2 "/5 -> Delay1/1
  Gateway In5/1 -> FIR Compiler 7.2 1/5, FIR Compiler 7.2 5/5, FIR Compiler 7.2 4/5, FIR Compiler 7.2 3/5, FIR Compiler 7.2 7/5, FIR Compiler 7.2 6/5, FIR Compiler 7.2 2/5, "FIR Compiler 7.2 "/5
  Shift/1 -> Y3/1
  Y3/1 -> Out4/1
  FIR Compiler 7.2 2/6 -> Terminator34/1
  FIR Compiler 7.2 3/1 -> Terminator24/1
  FIR Compiler 7.2 4/5 -> AddSub3/2, AddSub2/2
  FIR Compiler 7.2 3/7 -> Terminator29/1
  "FIR Compiler 7.2 "/6 -> Terminator10/1
  Y0/1 -> Out1/1
  X0/1 -> FIR Compiler 7.2 5/1, FIR Compiler 7.2 2/1, FIR Compiler 7.2 4/1, FIR Compiler 7.2 1/1
  FIR Compiler 7.2 5/4 -> Terminator15/1
  FIR Compiler 7.2 7/3 -> Terminator38/1
  FIR Compiler 7.2 3/2 -> Terminator25/1
  "FIR Compiler 7.2 "/3 -> Terminator8/1
  "FIR Compiler 7.2 "/7 -> Terminator11/1
  FIR Compiler 7.2 6/2 -> Terminator43/1
  H2/1 -> FIR Compiler 7.2 2/6, "FIR Compiler 7.2 "/6
  AddSub4/1 -> AddSub7/2
  AddSub8/1 -> FIR Compiler 7.2 7/6, FIR Compiler 7.2 5/6
  FIR Compiler 7.2 3/5 -> AddSub1/1
  In2/1 -> Gateway In2/1, Gateway In3/1, Gateway In4/1, Gateway In5/1, H3/1, H1/1, H2/1, H0/1
  FIR Compiler 7.2 2/4 -> Terminator33/1
  FIR Compiler 7.2 5/1 -> Terminator12/1
  Y2/1 -> Out3/1
  FIR Compiler 7.2 3/4 -> Terminator27/1
  H1/1 -> AddSub9/1, AddSub8/1
  FIR Compiler 7.2 4/4 -> Terminator21/1
  FIR Compiler 7.2 7/6 -> Terminator40/1
  In3/1 -> X1/1
  FIR Compiler 7.2 6/7 -> Terminator47/1
  Delay1/1 -> AddSub/2
  FIR Compiler 7.2 2/2 -> Terminator31/1
  AddSub6/1 -> Shift1/1
  FIR Compiler 7.2 4/2 -> Terminator19/1
  FIR Compiler 7.2 5/6 -> Terminator16/1
  "FIR Compiler 7.2 "/4 -> Terminator9/1
  FIR Compiler 7.2 1/4 -> Terminator3/1
  FIR Compiler 7.2 4/3 -> Terminator20/1
  FIR Compiler 7.2 6/1 -> Terminator42/1
  FIR Compiler 7.2 2/7 -> Terminator35/1
  FIR Compiler 7.2 2/3 -> Terminator32/1
  FIR Compiler 7.2 4/6 -> Terminator22/1
  AddSub/1 -> Y0/1
  FIR Compiler 7.2 4/7 -> Terminator23/1
  FIR Compiler 7.2 1/5 -> AddSub/1
  FIR Compiler 7.2 1/7 -> Terminator5/1
  FIR Compiler 7.2 3/6 -> Terminator28/1
  FIR Compiler 7.2 3/3 -> Terminator26/1
  FIR Compiler 7.2 5/7 -> Terminator17/1
  Delay2/1 -> AddSub1/2
  Reinterpret/1 -> FIR Compiler 7.2 6/6, FIR Compiler 7.2 4/6
  FIR Compiler 7.2 6/4 -> Terminator45/1
  H0/1 -> FIR Compiler 7.2 1/6, FIR Compiler 7.2 3/6
  FIR Compiler 7.2 2/5 -> Delay2/1
  H3/1 -> AddSub9/2, AddSub8/2
  AddSub9/1 -> Reinterpret/1
  "FIR Compiler 7.2 "/2 -> Terminator7/1
  FIR Compiler 7.2 7/4 -> Terminator39/1
  AddSub1/1 -> Y2/1
  FIR Compiler 7.2 1/1 -> Terminator/1
  AddSub2/1 -> AddSub6/1
  FIR Compiler 7.2 2/1 -> Terminator30/1
  FIR Compiler 7.2 5/3 -> Terminator14/1
